simulink model "smlnk"  (R2024a)
settings: Solver=ode4  StartTime=0.0  StopTime=20  FixedStep=0.0001  RelTol=1e-3
undefined symbols (not defined in the file or in its folder): Sample_Time
settings Model: Creator=loren  LastModifiedBy=alex1
settings RTWCC: GPUComputeCapability=3.5

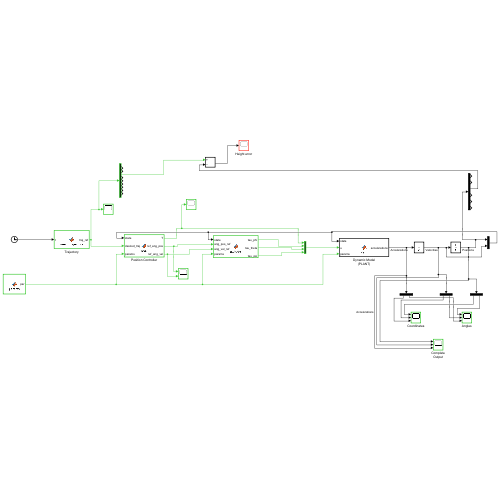
[thumbnail: Simulink's stored preview of the top-level diagram]
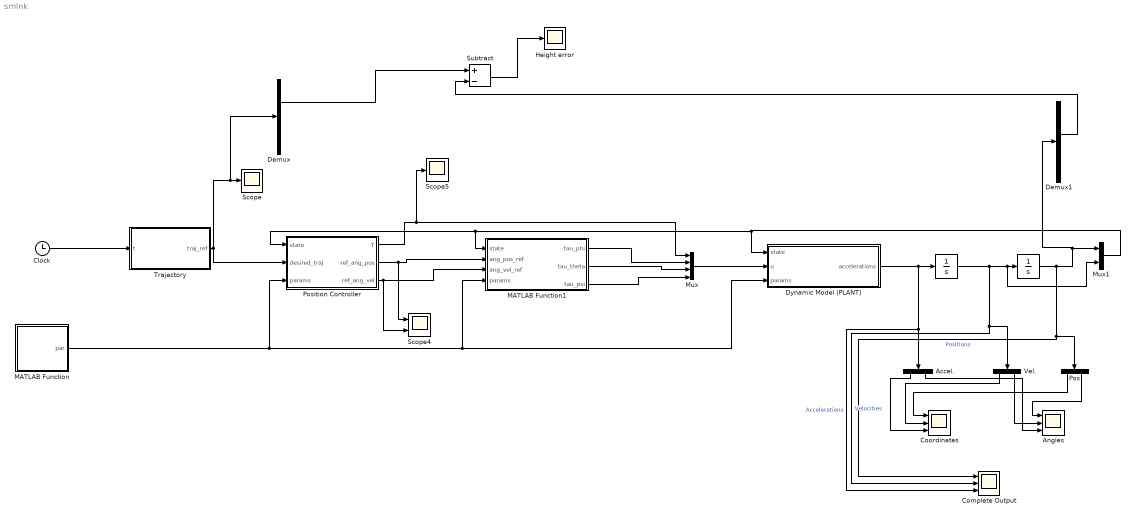
== system smlnk ==
  " " : Integrator  InitialCondition=[0 0 0 0 0 0]
  "  " : Integrator  InitialCondition=[0 0 0 0 0 0]
  Accel. : Demux  Tag=Accelerations  Outputs=2
  Angles : Scope  NumInputPorts=3
  Clock : Clock
  Complete Output : Scope  NumInputPorts=3
  Coordinates : Scope  NumInputPorts=3
  Demux : Demux  Outputs=9
  Demux1 : Demux  Outputs=6
  Dynamic Model (PLANT) : MATLAB Function  TreatAsAtomicUnit=on
  Height error : Scope
  MATLAB Function : MATLAB Function  TreatAsAtomicUnit=on  SystemSampleTime=Sample_Time
  MATLAB Function1 : MATLAB Function  TreatAsAtomicUnit=on  SystemSampleTime=Sample_Time
  Mux : Mux
  Mux1 : Mux  Inputs=2
  Pos : Demux  Outputs=2
  Position Controller : MATLAB Function  TreatAsAtomicUnit=on  SystemSampleTime=Sample_Time
  Scope : Scope
  Scope4 : Scope  NumInputPorts=2
  Scope5 : Scope
  Subtract : Sum  Inputs=+-
  Trajectory : MATLAB Function  TreatAsAtomicUnit=on  SystemSampleTime=Sample_Time
  Vel. : Demux  Outputs=2
  wires:
  Trajectory/1(traj_ref) -> Demux/1, Scope/1, Position Controller/2(desired_traj)
  MATLAB Function/1(par) -> Dynamic Model (PLANT)/3(params), MATLAB Function1/4(params), Position Controller/3(params)
  Position Controller/2(ref_ang_pos) -> Scope4/1, MATLAB Function1/2(ang_pos_ref)
  Position Controller/3(ref_ang_vel) -> Scope4/2, MATLAB Function1/3(ang_vel_ref)
  MATLAB Function1/1(tau_phi) -> Mux/2
  MATLAB Function1/2(tau_theta) -> Mux/3
  MATLAB Function1/3(tau_psi) -> Mux/4
  Position Controller/1(T) -> Scope5/1, Mux/1
  Mux/1 -> Dynamic Model (PLANT)/2(u)
  Dynamic Model (PLANT)/1(accelerations) -> " "/1, Accel./1, Complete Output/3  "Accelerations"
  " "/1 -> "  "/1, Mux1/2, Vel./1, Complete Output/2  "Velocities"
  Mux1/1 -> Dynamic Model (PLANT)/1(state), Position Controller/1(state), MATLAB Function1/1(state)
  Demux/3 -> Subtract/1
  Demux1/3 -> Subtract/2
  Subtract/1 -> Height error/1
  Clock/1 -> Trajectory/1(t)
  "  "/1 -> Pos/1, Complete Output/1, Demux1/1, Mux1/1  "Positions"
  Pos/1 -> Coordinates/1
  Vel./1 -> Coordinates/2
  Accel./1 -> Coordinates/3
  Pos/2 -> Angles/1
  Vel./2 -> Angles/2
  Accel./2 -> Angles/3

== matlab function smlnk/Trajectory ==
  data: traj_ref output; t input
function traj_ref = linear_trajectory(t)

% Chiama la funzione per generare la traiettoria
[pos, vel, acc] = only_linear_trajectory(t);
traj_ref = [pos, vel, acc];

== matlab function smlnk/Position Controller ==
  data: state input; desired_traj input; T output; ref_ang_pos output; ref_ang_vel output; params input
function [T,ref_ang_pos,ref_ang_vel] = pos(state,desired_traj,params)

[T,ref_ang_pos,ref_ang_vel] = position_control(desired_traj,state,params);

== matlab function smlnk/MATLAB Function ==
  data: par output
function par = params()

[m,g,Ix,Iy,Iz,Kp_pos,Kd_pos,Ki_pos,Kp_ang,Kd_ang,Ki_ang,dt] = model_n_control_param();
par = [m,g,Ix,Iy,Iz,Kp_pos,Kd_pos,Ki_pos,Kp_ang,Kd_ang,Ki_ang,dt];

== matlab function smlnk/MATLAB Function1 ==
  data: state input; ang_pos_ref input; tau_phi output; ang_vel_ref input; params input; tau_theta output; tau_psi output
function [tau_phi,tau_theta,tau_psi] = attitude(state,ang_pos_ref,ang_vel_ref,params)

[tau_phi,tau_theta,tau_psi] = attitude_control(ang_pos_ref,ang_vel_ref,state,params)

== matlab function smlnk/Dynamic Model (PLANT) ==
  data: state input; u input; accelerations output; params input
function accelerations = dyn(state,u,params)

accelerations = dynamic_model(state, u, params);
